simulink model "Digital Protection - Instantaneous Overcurrent Element SLG Simulink"  (R2024b)
settings: Solver=ode4  StartTime=0.0  StopTime=1  FixedStep=1e-5  RelTol=1e-4
undefined symbols (not defined in the file): D1, Delta, dspblkCoreblockFVToolHelper, gcbh, rvar
libraries: spsThreePhaseBreakerLib x6, dspfdesign x6, powerlib_extras x6, simulink_extras x6, spsLoadFlowBusLib x4, spsThreePhaseVIMeasurementLib x4, spsDistributedParametersLineLib x3, spsThreePhaseSeriesRLCLoadLib x3, spsGroundLib x3, spsThreePhaseSeriesRLCBranchLib x2, spsSeriesRLCBranchLib x2, spsThreePhaseTransformerTwoWindingsLib x1
(part 1 of 2)
settings Model: Creator=The MathWorks, Inc.  LastModifiedBy=ECDG
settings SolverCC: AlgebraicLoopSolver=TrustRegion  EnableFixedStepZeroCrossing=on
settings DataIOCC: SaveFormat=Array  ReturnWorkspaceOutputs=off  SignalLoggingName=sigsOut
settings OptimizationCC: BlockReduction=off  BooleanDataType=off  ReuseModelBlockBuffer=off  ExpressionDepthLimit=2147483647  InitFltsAndDblsToZero=on  LifeSpan=inf
settings DebuggingCC: UnderspecifiedInitializationDetection=Classic  MergeDetectMultiDrivingBlocksExec=none  CheckExecutionContextPreStartOutputMsg=on  SignalResolutionControl=TryResolveAllWithWarning  MultiTaskDSMMsg=warning  MultiTaskCondExecSysMsg=none  FcnCallInpInsideContextMsg=warning  UnconnectedInputMsg=warning  UnconnectedOutputMsg=warning  UnconnectedLineMsg=warning  StateNameClashWarn=warning  SFUnexpectedBacktrackingDiag=warning  SFNoUnconditionalDefaultTransitionDiag=warning  SFExecutionAtInitializationDiag=none  ArithmeticOperatorsInVariantConditions=warning
settings HardwareCC: ProdBitPerPointer=32  ProdBitPerSizeT=32  ProdBitPerPtrDiffT=32  ProdLargestAtomicFloat=None  ProdIntDivRoundTo=Undefined  ProdEndianess=Unspecified  ProdWordSize=32  ProdHWDeviceType=32-bit Generic  TargetUnknown=on
settings ModelReferenceCC: EnableRefExpFcnMdlSchedulingChecks=on  PropagateSignalLabelsOutOfModel=off
settings SFSimCC: SimUseLocalCustomCode=off  CustomCodeUndefinedFunction=UseInterfaceOnly
settings RTWCC: RTWUseLocalCustomCode=off  GPUComputeCapability=3.5  DLArmComputeVersion=19.05
settings CodeAppCC: StateflowObjectComments=on
settings GRTTargetCC: TargetLangStandard=C89/C90 (ANSI)  CombineOutputUpdateFcns=off  GRTInterface=on
settings ConfigComp: CovMetricSettings=dw  CovSaveCumulativeToWorkspaceVar=on  CovSaveSingleToWorkspaceVar=on  CovExternalEMLEnable=off  CovSFcnEnable=off
settings SimscapeCC: SimscapeNormalizeSystem=off

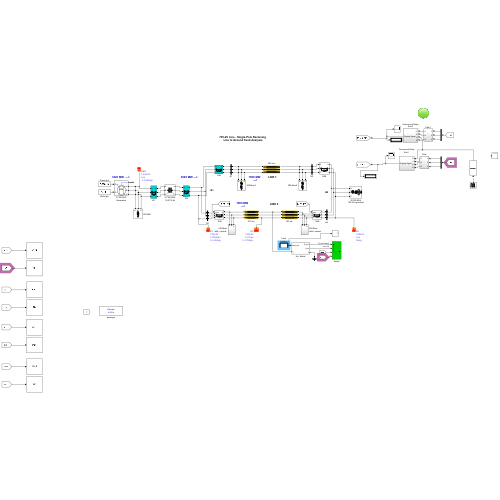
[thumbnail: Simulink's stored preview of the top-level diagram]
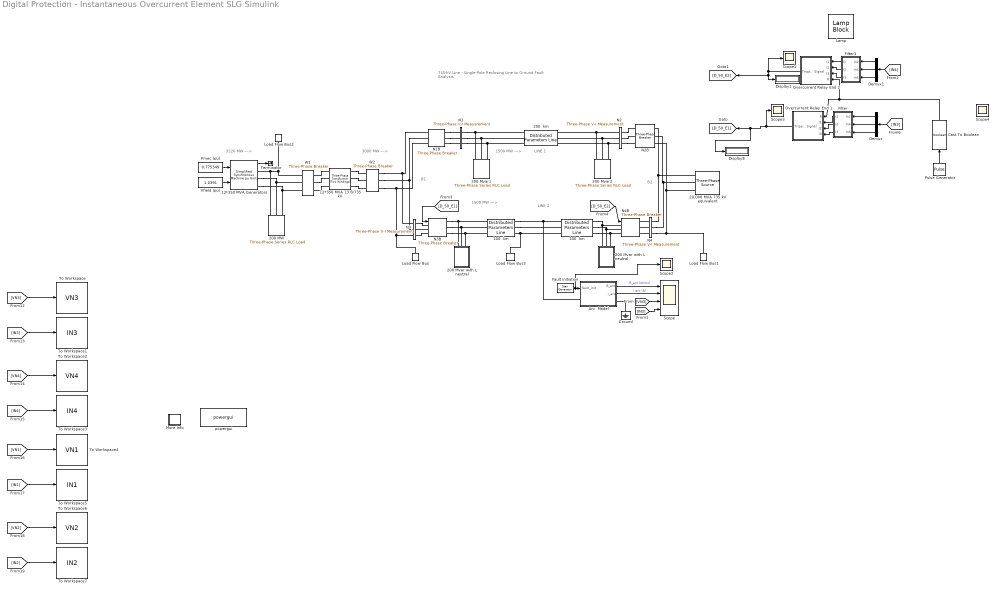
== system Digital Protection - Instantaneous Overcurrent Element SLG Simulink ==
  note: 735-kV Line - Single-Pole Reclosing
      | Line to Ground Fault Analysis
  note: LINE 1
  note: LINE 2
  note: B1
  note: B2
  note: 1500 MW
      |   --->
  note: 1500 MW
      |   --->
  note: 3220 MW --->
  note: 3000 MW --->
  "  N3B" : spsThreePhaseBreakerLib/Three-Phase Breaker  InitialState=closed  SwitchA=on  SwitchB=off  SwitchC=off  SwitchTimes=[0.4]  External=on  BreakerResistance=0.001  SnubberResistance=1e5  SnubberCapacitance=inf  Measurements=None
      settings: AttributesFormatString=\n
  "  N4B" : spsThreePhaseBreakerLib/Three-Phase Breaker  InitialState=closed  SwitchA=on  SwitchB=off  SwitchC=off  SwitchTimes=[0.2]  External=on  BreakerResistance=0.001  SnubberResistance=1e5  SnubberCapacitance=inf  Measurements=None
      settings: AttributesFormatString=\n
  " N1B" : spsThreePhaseBreakerLib/Three-Phase Breaker  InitialState=closed  SwitchA=off  SwitchB=off  SwitchC=off  SwitchTimes="[4/60  34/60]"  External=off  BreakerResistance=0.001  SnubberResistance=1e5  SnubberCapacitance=inf  Measurements=None
      settings: AttributesFormatString=\n
  " W2" : spsThreePhaseBreakerLib/Three-Phase Breaker  InitialState=closed  SwitchA=off  SwitchB=off  SwitchC=off  SwitchTimes="[4/60  34/60]"  External=off  BreakerResistance=0.001  SnubberResistance=1e5  SnubberCapacitance=inf  Measurements=Breaker voltages and currents
      settings: AttributesFormatString=\n
  "100  km " : spsDistributedParametersLineLib/Distributed Parameters Line  Phases=3  Length=100  Frequency=60  Resistance=[0.01165 0.2676]  Inductance="[0.8679e-3  3.008e-3]"  Capacitance="[13.41e-9  8.57e-9]"  x1=[-0.00051 -3.77922811047225e-08 0 0;-0.0005 -3.76584518295274e-08 0 0;-0.00049 -3.75240873443748e-08 0 0;-0.00048 -3.73891895588812e-08 0 0;-0.00047 -3.72537603902428e-08 0 0;-0.00046 -3.71178017632078e-08 0 0;-0.00045 -3.69813156100494e-08 0 0;-0.00044 -3.68443038705378e-08 0 0;-0.00043 -3.67067684919131e-08 0 0;-0.00042 -3.65687114288575e-08 0 0;-0.00041 -3.64301346434675e-08 0 0;-0.0004 -3.6291040105226e-08 0 0;-0.00039 -3.61514297909741e-08 0 0;-0.00038 -3.60113056848835e-08 0 0;-0.00037 -3.58706697784279e-08 0 0;-0.00036 -3.57295240703548e-08 0 0;-0.00035 -3.55878705666572e-08 395978.931287506 -613583.344384587;-0.00034 -3.54457112805449e-08 398289.270800667 -612086.189257274;-0.00033 -3.53030482324161e-08 400593.949741675 -610580.335030357;-0.00032 -3.51598834498283e-08 402892.93535594 -609065.803105355;-0.00031 -3.50162189674702e-08 405186.194969788 -607542.615007121;-0.0003 -3.4872056827132e-08 407473.695990923 -606010.792383529;-0.00029 -3.47273990776767e-08 409755.405908894 -604470.35700517;-0.00028 -3.45822477750113e-08 412031.292295551 -602921.330765038;-0.00027 -3.4436604982057e-08 414301.32280551 -601363.735678227;-0.00026 -3.42904727687203e-08 416565.465176615 -599797.593881611;-0.00025 -3.41438532118635e-08 418823.687230389 -598222.92763353;-0.00024 -3.39967483952749e-08 421075.9568725 -596639.759313478;-0.00023 -3.38491604096396e-08 423322.242093209 -595048.11142178;-0.00022 -3.37010913525096e-08 425562.510967832 -593448.006579278;-0.00021 -3.35525433282739e-08 427796.73165719 -591839.467527001;-0.0002 -3.34035184481288e-08 430024.87240806 -590222.517125851;-0.00019 -3.32540188300477e-08 432246.901553632 -588597.178356272;-0.00018 -3.3104046598751e-08 434462.787513951 -586963.474317926;-0.00017 -3.29536038856763e-08 436672.498796374 -585321.428229363;-0.00016 -3.28026928289473e-08 438876.003996012 -583671.063427693;-0.00015 -3.26513155733443e-08 441073.271796179 -582012.403368252;-0.00014 -3.24994742702731e-08 443264.270968836 -580345.471624272;-0.00013 -3.23471710777348e-08 445448.970375035 -578670.291886542;-0.00012 -3.21944081602949e-08 447627.338965361 -576986.887963075;-0.00011 -3.20411876890525e-08 449799.345780374 -575295.283778767;-0.0001 -3.18875118416097e-08 451964.959951051 -573595.503375057;-9e-05 -3.17333828020404e-08 454124.15069922 -571887.570909587;-8e-05 -3.15788027608595e-08 456276.887338002 -570171.510655858;-7e-05 -3.14237739149916e-08 458423.139272243 -568447.347002886;-6e-05 -3.12682984677396e-08 460562.875998953 -566715.104454851;-5e-05 -3.11123786287539e-08 462696.067107737 -564974.807630755;-4e-05 -3.09560166140004e-08 464822.682281227 -563226.481264068;-3e-05 -3.07992146457295e-08 466942.691295515 -561470.150202377;-2e-05 -3.06419749524443e-08 469056.064020578 -559705.839407035;-1e-05 -3.04842997688688e-08 471162.770420715 -557933.573952803]  x2=[-0.00051 -2.56040253138392e-08 0 0;-0.0005 -2.55064962507539e-08 0 0;-0.00049 -2.54086046838981e-08 0 0;-0.00048 -2.53103520045277e-08 0 0;-0.00047 -2.52117396090307e-08 0 0;-0.00046 -2.51127688989075e-08 0 0;-0.00045 -2.5013441280751e-08 0 0;-0.00044 -2.49137581662265e-08 0 0;-0.00043 -2.48137209720518e-08 0 0;-0.00042 -2.47133311199767e-08 0 0;-0.00041 -2.46125900367634e-08 0 0;-0.0004 -2.45114991541655e-08 0 0;-0.00039 -2.44100599089083e-08 0 0;-0.00038 -2.4308273742668e-08 0 0;-0.00037 -2.42061421020513e-08 0 0;-0.00036 -2.41036664385749e-08 0 0;-0.00035 -2.40008482086449e-08 340840.176223379 -651975.861370538;-0.00034 -2.38976888735358e-08 343295.642553621 -650686.299268294;-0.00033 -2.37941898993701e-08 345746.229892895 -649387.48947344;-0.00032 -2.36903527570974e-08 348191.903412932 -648079.450444938;-0.00031 -2.35861789224733e-08 350632.628355296 -646762.200772918;-0.0003 -2.34816698760386e-08 353068.370031884 -645435.759178413;-0.00029 -2.33768271030981e-08 355499.093825416 -644100.144513095;-0.00028 -2.32716520936998e-08 357924.765189925 -642755.375759005;-0.00027 -2.31661463426133e-08 360345.349651252 -641401.472028282;-0.00026 -2.30603113493089e-08 362760.812807534 -640038.452562896;-0.00025 -2.29541486179361e-08 365171.120329694 -638666.336734371;-0.00024 -2.28476596573023e-08 367576.237961925 -637285.14404351;-0.00023 -2.27408459808514e-08 369976.131522183 -635894.894120118;-0.00022 -2.26337091066421e-08 372370.766902668 -634495.606722723;-0.00021 -2.25262505573265e-08 374760.110070311 -633087.301738298;-0.0002 -2.24184718601286e-08 377144.127067255 -631669.999181973;-0.00019 -2.23103745468221e-08 379522.784011344 -630243.719196755;-0.00018 -2.22019601537092e-08 381896.047096597 -628808.482053238;-0.00017 -2.20932302215983e-08 384263.882593691 -627364.308149322;-0.00016 -2.19841862957825e-08 386626.256850443 -625911.218009912;-0.00015 -2.18748299260173e-08 388983.136292286 -624449.232286636;-0.00014 -2.17651626664989e-08 391334.487422747 -622978.371757548;-0.00013 -2.16551860758416e-08 393680.27682392 -621498.657326831;-0.00012 -2.15449017170563e-08 396020.471156946 -620010.110024504;-0.00011 -2.14343111575279e-08 398355.037162483 -618512.751006117;-0.0001 -2.13234159689929e-08 400683.941661182 -617006.601552457;-9e-05 -2.12122177275176e-08 403007.151554153 -615491.683069241;-8e-05 -2.1100718013475e-08 405324.633823443 -613968.017086816;-7e-05 -2.09889184115228e-08 407636.355532497 -612435.625259845;-6e-05 -2.0876820510581e-08 409942.283826634 -610894.529367011;-5e-05 -2.07644259038087e-08 412242.385933509 -609344.751310696;-4e-05 -2.06517361885822e-08 414536.629163579 -607786.313116677;-3e-05 -2.05387529664718e-08 416824.980910569 -606219.23693381;-2e-05 -2.0425477843219e-08 419107.408651936 -604643.545033717;-1e-05 -2.03119124287142e-08 421383.87994933 -603059.259810467]  x3=[-0.00051 3.42496863435419e-11 0 0;-0.0005 3.47494854439e-11 0 0;-0.00049 3.52487906771517e-11 0 0;-0.00048 3.57475949470645e-11 0 0;-0.00047 3.62458911645256e-11 0 0;-0.00046 3.67436722476428e-11 0 0;-0.00045 3.72409311218451e-11 0 0;-0.00044 3.77376607199831e-11 0 0;-0.00043 3.82338539824298e-11 0 0;-0.00042 3.87295038571805e-11 0 0;-0.00041 3.92246032999535e-11 0 0;-0.0004 3.97191452742897e-11 0 0;-0.00039 4.0213122751653e-11 0 0;-0.00038 4.07065287115301e-11 0 0;-0.00037 4.119935614153e-11 0 0;-0.00036 4.16915980374842e-11 0 0;-0.00035 4.21832474035457e-11 164.000176487801 -861.324068209358;-0.00034 4.26742972522888e-11 167.246078376088 -860.699738770174;-0.00033 4.31647406048081e-11 170.4896033274 -860.063176882539;-0.00032 4.36545704908181e-11 173.73070524407 -859.414391593406;-0.00031 4.41437799487517e-11 176.969338062865 -858.75339212345;-0.0003 4.46323620258598e-11 180.205455755643 -858.080187866937;-0.00029 4.51203097783096e-11 183.439012330009 -857.39478839159;-0.00028 4.56076162712833e-11 186.669961829966 -856.697203438451;-0.00027 4.60942745790771e-11 189.898258336571 -855.987442921748;-0.00026 4.65802777851993e-11 193.123855968584 -855.265516928748;-0.00025 4.70656189824684e-11 196.346708883124 -854.531435719618;-0.00024 4.75502912731118e-11 199.566771276315 -853.785209727276;-0.00023 4.80342877688633e-11 202.783997383945 -853.026849557246;-0.00022 4.85176015910616e-11 205.998341482108 -852.256365987505;-0.00021 4.90002258707472e-11 209.209757887861 -851.473769968328;-0.0002 4.9482153748761e-11 212.418200959867 -850.679072622139;-0.00019 4.9963378375841e-11 215.623625099048 -849.872285243346;-0.00018 5.044389291272e-11 218.825984749233 -849.053419298182;-0.00017 5.0923690530223e-11 222.025234397802 -848.222486424545;-0.00016 5.14027644093637e-11 225.221328576336 -847.379498431832;-0.00015 5.18811077414418e-11 228.414221861263 -846.524467300767;-0.00014 5.23587137281398e-11 231.603868874501 -845.657405183235;-0.00013 5.28355755816194e-11 234.790224284105 -844.778324402109;-0.00012 5.33116865246182e-11 237.973242804914 -843.887237451071;-0.00011 5.37870397905458e-11 241.152879199187 -842.98415699444;-0.0001 5.426162862358e-11 244.329088277253 -842.069095866989;-9e-05 5.47354462787631e-11 247.501824898151 -841.142067073761;-8e-05 5.52084860220974e-11 250.671043970271 -840.203083789887;-7e-05 5.56807411306411e-11 253.836700451994 -839.252159360399;-6e-05 5.61522048926036e-11 256.998749352335 -838.289307300037;-5e-05 5.66228706074415e-11 260.15714573158 -837.314541293061;-4e-05 5.70927315859529e-11 263.311844701925 -836.327875193052;-3e-05 5.75617811503735e-11 266.462801428114 -835.329323022721;-2e-05 5.80300126344706e-11 269.609971128078 -834.318898973704;-1e-05 5.84974193836385e-11 272.753309073569 -833.296617406363]  x4=[-0.00051 -1.51149043943084e-10 0 0;-0.0005 -1.51308414634417e-10 0 0;-0.00049 -1.51465634898256e-10 0 0;-0.00048 -1.51620702500153e-10 0 0;-0.00047 -1.51773615236255e-10 0 0;-0.00046 -1.51924370933332e-10 0 0;-0.00045 -1.52072967448813e-10 0 0;-0.00044 -1.52219402670812e-10 0 0;-0.00043 -1.52363674518161e-10 0 0;-0.00042 -1.52505780940437e-10 0 0;-0.00041 -1.52645719917994e-10 0 0;-0.0004 -1.52783489461988e-10 0 0;-0.00039 -1.52919087614411e-10 0 0;-0.00038 -1.5305251244811e-10 0 0;-0.00037 -1.53183762066826e-10 0 0;-0.00036 -1.53312834605209e-10 0 0;-0.00035 -1.53439728228854e-10 2402.72875516981 -4282.32087607898;-0.00034 -1.53564441134322e-10 2418.85568395253 -4273.23238215375;-0.00033 -1.53686971549165e-10 2434.94823544183 -4264.08315613756;-0.00032 -1.53807317731955e-10 2451.00618092693 -4254.87332806114;-0.00031 -1.53925477972307e-10 2467.02929218889 -4245.60302881654;-0.0003 -1.54041450590902e-10 2483.01734150382 -4236.27239015525;-0.00029 -1.54155233939513e-10 2498.97010164616 -4226.88154468627;-0.00028 -1.54266826401026e-10 2514.88734589186 -4217.43062587432;-0.00027 -1.54376226389465e-10 2530.76884802167 -4207.91976803788;-0.00026 -1.54483432350015e-10 2546.61438232428 -4198.34910634727;-0.00025 -1.54588442759041e-10 2562.42372359957 -4188.7187768228;-0.00024 -1.54691256124114e-10 2578.19664716181 -4179.02891633276;-0.00023 -1.54791870984027e-10 2593.93292884284 -4169.27966259151;-0.00022 -1.5489028590882e-10 2609.63234499527 -4159.47115415754;-0.00021 -1.54986499499801e-10 2625.29467249564 -4149.60353043146;-0.0002 -1.5508051038956e-10 2640.91968874761 -4139.67693165403;-0.00019 -1.55172317241994e-10 2656.50717168512 -4129.69149890421;-0.00018 -1.55261918752327e-10 2672.05689977552 -4119.6473740971;-0.00017 -1.5534931364712e-10 2687.56865202276 -4109.54469998194;-0.00016 -1.554345006843e-10 2703.04220797051 -4099.3836201401;-0.00015 -1.55517478653171e-10 2718.47734770529 -4089.16427898301;-0.00014 -1.5559824637443e-10 2733.87385185959 -4078.88682175012;-0.00013 -1.55676802700192e-10 2749.23150161502 -4068.55139450686;-0.00012 -1.55753146513995e-10 2764.55007870536 -4058.15814414253;-0.00011 -1.55827276730826e-10 2779.82936541975 -4047.70721836821;-0.0001 -1.55899192297131e-10 2795.06914460568 -4037.1987657147;-9e-05 -1.55968892190829e-10 2810.26919967217 -4026.63293553036;-8e-05 -1.56036375421331e-10 2825.42931459278 -4016.00987797904;-7e-05 -1.56101641029551e-10 2840.54927390874 -4005.32974403789;-6e-05 -1.5616468808792e-10 2855.62886273193 -3994.59268549527;-5e-05 -1.562255157004e-10 2870.66786674804 -3983.79885494852;-4e-05 -1.56284123002496e-10 2885.66607221953 -3972.9484058019;-3e-05 -1.56340509161269e-10 2900.62326598869 -3962.04149226428;-2e-05 -1.56394673375345e-10 2915.5392354807 -3951.07826934705;-1e-05 -1.56446614874933e-10 2930.41376870661 -3940.05889286189]  x5=0.000507725910309884  V1=ones(3,3)  V2=ones(3,3)  I1=ones(3,3)  I2=ones(3,3)  nHarmo=1  Measurements=None  Decoupling=off  VsMag0=0  VrMag0=0  VsAngle0=0  VrAngle0=0  IsMag0=0  IrMag0=0  IsAngle0=0  IrAngle0=0
      settings: AttributesFormatString=\n
  "100  km  " : spsDistributedParametersLineLib/Distributed Parameters Line  Phases=3  Length=100  Frequency=60  Resistance=[0.01165 0.2676]  Inductance="[0.8679e-3  3.008e-3]"  Capacitance="[13.41e-9  8.57e-9]"  x1=[-0.00051 -2.56040253138392e-08 0 0;-0.0005 -2.55064962507539e-08 0 0;-0.00049 -2.54086046838981e-08 0 0;-0.00048 -2.53103520045277e-08 0 0;-0.00047 -2.52117396090307e-08 0 0;-0.00046 -2.51127688989075e-08 0 0;-0.00045 -2.5013441280751e-08 0 0;-0.00044 -2.49137581662265e-08 0 0;-0.00043 -2.48137209720518e-08 0 0;-0.00042 -2.47133311199767e-08 0 0;-0.00041 -2.46125900367634e-08 0 0;-0.0004 -2.45114991541655e-08 0 0;-0.00039 -2.44100599089083e-08 0 0;-0.00038 -2.4308273742668e-08 0 0;-0.00037 -2.42061421020513e-08 0 0;-0.00036 -2.41036664385749e-08 0 0;-0.00035 -2.40008482086449e-08 340840.176223379 -651975.861370538;-0.00034 -2.38976888735358e-08 343295.642553621 -650686.299268294;-0.00033 -2.37941898993701e-08 345746.229892895 -649387.48947344;-0.00032 -2.36903527570974e-08 348191.903412932 -648079.450444938;-0.00031 -2.35861789224733e-08 350632.628355296 -646762.200772918;-0.0003 -2.34816698760386e-08 353068.370031884 -645435.759178413;-0.00029 -2.33768271030981e-08 355499.093825416 -644100.144513095;-0.00028 -2.32716520936998e-08 357924.765189925 -642755.375759005;-0.00027 -2.31661463426133e-08 360345.349651252 -641401.472028282;-0.00026 -2.30603113493089e-08 362760.812807534 -640038.452562896;-0.00025 -2.29541486179361e-08 365171.120329694 -638666.336734371;-0.00024 -2.28476596573023e-08 367576.237961925 -637285.14404351;-0.00023 -2.27408459808514e-08 369976.131522183 -635894.894120118;-0.00022 -2.26337091066421e-08 372370.766902668 -634495.606722723;-0.00021 -2.25262505573265e-08 374760.110070311 -633087.301738298;-0.0002 -2.24184718601286e-08 377144.127067255 -631669.999181973;-0.00019 -2.23103745468221e-08 379522.784011344 -630243.719196755;-0.00018 -2.22019601537092e-08 381896.047096597 -628808.482053238;-0.00017 -2.20932302215983e-08 384263.882593691 -627364.308149322;-0.00016 -2.19841862957825e-08 386626.256850443 -625911.218009912;-0.00015 -2.18748299260173e-08 388983.136292286 -624449.232286636;-0.00014 -2.17651626664989e-08 391334.487422747 -622978.371757548;-0.00013 -2.16551860758416e-08 393680.27682392 -621498.657326831;-0.00012 -2.15449017170563e-08 396020.471156946 -620010.110024504;-0.00011 -2.14343111575279e-08 398355.037162483 -618512.751006117;-0.0001 -2.13234159689929e-08 400683.941661182 -617006.601552457;-9e-05 -2.12122177275176e-08 403007.151554153 -615491.683069241;-8e-05 -2.1100718013475e-08 405324.633823443 -613968.017086816;-7e-05 -2.09889184115228e-08 407636.355532497 -612435.625259845;-6e-05 -2.0876820510581e-08 409942.283826634 -610894.529367011;-5e-05 -2.07644259038087e-08 412242.385933509 -609344.751310696;-4e-05 -2.06517361885822e-08 414536.629163579 -607786.313116677;-3e-05 -2.05387529664718e-08 416824.980910569 -606219.23693381;-2e-05 -2.0425477843219e-08 419107.408651936 -604643.545033717;-1e-05 -2.03119124287142e-08 421383.87994933 -603059.259810467]  x2=[-0.00051 -1.18539215505797e-08 0 0;-0.0005 -1.17942402554783e-08 0 0;-0.00049 -1.17343913381163e-08 0 0;-0.00048 -1.16743756490792e-08 0 0;-0.00047 -1.16141940413229e-08 0 0;-0.00046 -1.15538473701611e-08 0 0;-0.00045 -1.14933364932537e-08 0 0;-0.00044 -1.14326622705942e-08 0 0;-0.00043 -1.13718255644975e-08 0 0;-0.00042 -1.1310827239588e-08 0 0;-0.00041 -1.12496681627868e-08 0 0;-0.0004 -1.11883492032999e-08 0 0;-0.00039 -1.11268712326053e-08 0 0;-0.00038 -1.10652351244411e-08 0 0;-0.00037 -1.10034417547928e-08 0 0;-0.00036 -1.0941492001881e-08 0 0;-0.00035 -1.08793867461488e-08 280454.28762092 -679398.727325685;-0.00034 -1.08171268702493e-08 283013.563488485 -678336.617298876;-0.00033 -1.07547132590333e-08 285568.817106861 -677264.866607234;-0.00032 -1.06921467995362e-08 288120.012160238 -676183.490482708;-0.00031 -1.0629428380966e-08 290667.112390487 -675092.504294046;-0.0003 -1.05665588946902e-08 293210.081597675 -673991.923546578;-0.00029 -1.05035392342234e-08 295748.883640582 -672881.763881991;-0.00028 -1.04403702952144e-08 298283.482437211 -671762.041078112;-0.00027 -1.03770529754337e-08 300813.841965302 -670632.77104868;-0.00026 -1.03135881747606e-08 303339.926262846 -669493.969843123;-0.00025 -1.02499767951703e-08 305861.699428593 -668345.653646326;-0.00024 -1.01862197407214e-08 308379.125622564 -667187.838778404;-0.00023 -1.01223179175427e-08 310892.169066562 -666020.541694469;-0.00022 -1.00582722338206e-08 313400.794044676 -664843.778984397;-0.00021 -9.99408359978607e-09 315904.964903792 -663657.56737259;-0.0002 -9.92975292770159e-09 318404.6460541 -662461.923717741;-0.00019 -9.86528113184844e-09 320899.801969597 -661256.865012593;-0.00018 -9.80066912851356e-09 323390.397188594 -660042.408383698;-0.00017 -9.73591783597653e-09 325876.396314221 -658818.571091172;-0.00016 -9.67102817449654e-09 328357.764014927 -657585.370528453;-0.00015 -9.60600106629932e-09 330834.465024985 -656342.824222049;-0.00014 -9.54083743556401e-09 333306.464144991 -655090.949831296;-0.00013 -9.47553820841005e-09 335773.726242367 -653829.765148098;-0.00012 -9.410104312884e-09 338236.216251855 -652559.288096681;-0.00011 -9.34453667894634e-09 340693.899176022 -651279.536733337;-0.0001 -9.2788362384583e-09 343146.740085755 -649990.529246166;-9e-05 -9.21300392516855e-09 345594.704120754 -648692.283954816;-8e-05 -9.1470406747e-09 348037.756490031 -647384.819310228;-7e-05 -9.08094742453643e-09 350475.862472406 -646068.153894367;-6e-05 -9.01472511400924e-09 352908.987416994 -644742.306419965;-5e-05 -8.94837468428403e-09 355337.096743706 -643407.295730247;-4e-05 -8.88189707834729e-09 357760.155943732 -642063.140798672;-3e-05 -8.81529324099293e-09 360178.130580038 -640709.860728656;-2e-05 -8.74856411880893e-09 362590.986287852 -639347.474753305;-1e-05 -8.6817106601638e-09 364998.688775155 -637976.002235138]  x3=[-0.00051 6.32300703573828e-11 0 0;-0.0005 6.37254256125662e-11 0 0;-0.00049 6.42198751883951e-11 0 0;-0.00048 6.47134120576465e-11 0 0;-0.00047 6.52060292060691e-11 0 0;-0.00046 6.56977196324828e-11 0 0;-0.00045 6.61884763488782e-11 0 0;-0.00044 6.66782923805162e-11 0 0;-0.00043 6.71671607660268e-11 0 0;-0.00042 6.76550745575079e-11 0 0;-0.00041 6.81420268206248e-11 0 0;-0.0004 6.86280106347078e-11 0 0;-0.00039 6.91130190928512e-11 0 0;-0.00038 6.95970453020112e-11 0 0;-0.00037 7.00800823831041e-11 0 0;-0.00036 7.05621234711037e-11 0 0;-0.00035 7.10431617151392e-11 267.626302043254 -825.665681968738;-0.00034 7.15231902785922e-11 270.737031817784 -824.650940062222;-0.00033 7.20022023391944e-11 273.843913819813 -823.624478040479;-0.00032 7.24801910891242e-11 276.946903893672 -822.586310491806;-0.00031 7.29571497351032e-11 280.045957939003 -821.536452170861;-0.0003 7.34330714984936e-11 283.141031911389 -820.474917998456;-0.00029 7.39079496153934e-11 286.232081822977 -819.401723061341;-0.00028 7.43817773367335e-11 289.319063743106 -818.316882611991;-0.00027 7.48545479283732e-11 292.40193379893 -817.22041206839;-0.00026 7.5326254671196e-11 295.480648176041 -816.112327013812;-0.00025 7.57968908612048e-11 298.555163119094 -814.992643196598;-0.00024 7.62664498096176e-11 301.625434932426 -813.861376529934;-0.00023 7.67349248429625e-11 304.691419980678 -812.718543091623;-0.00022 7.72023093031721e-11 307.753074689415 -811.564159123858;-0.00021 7.76685965476789e-11 310.810355545749 -810.39824103299;-0.0002 7.81337799495088e-11 313.863219098949 -809.220805389296;-0.00019 7.85978528973762e-11 316.911621961069 -808.031868926743;-0.00018 7.90608087957771e-11 319.955520807555 -806.83144854275;-0.00017 7.95226410650835e-11 322.994872377866 -805.619561297947;-0.00016 7.99833431416366e-11 326.029633476091 -804.396224415936;-0.00015 8.04429084778401e-11 329.059760971555 -803.16145528304;-0.00014 8.09013305422533e-11 332.085211799441 -801.915271448062;-0.00013 8.1358602819684e-11 335.105942961394 -800.657690622033;-0.00012 8.18147188112809e-11 338.12191152614 -799.388730677961;-0.00011 8.22696720346262e-11 341.133074630088 -798.108409650574;-0.0001 8.27234560238275e-11 344.139389477945 -796.816745736069;-9e-05 8.317606432961e-11 347.140813343324 -795.513757291849;-8e-05 8.36274905194076e-11 350.137303569347 -794.199462836264;-7e-05 8.40777281774551e-11 353.128817569255 -792.873881048347;-6e-05 8.45267709048787e-11 356.115312827014 -791.537030767551;-5e-05 8.49746123197872e-11 359.096746897913 -790.188930993475;-4e-05 8.5421246057363e-11 362.073077409177 -788.829600885603;-3e-05 8.58666657699519e-11 365.044262060561 -787.459059763024;-2e-05 8.63108651271539e-11 368.010258624953 -786.077327104161;-1e-05 8.67538378159128e-11 370.971024948977 -784.684422546493]  x4=[-0.00051 -1.32243517909503e-10 0 0;-0.0005 -1.3251038312282e-10 0 0;-0.00049 -1.32775365070281e-10 0 0;-0.00048 -1.33038459985904e-10 0 0;-0.00047 -1.3329966413053e-10 0 0;-0.00046 -1.3355897379187e-10 0 0;-0.00045 -1.33816385284558e-10 0 0;-0.00044 -1.34071894950208e-10 0 0;-0.00043 -1.34325499157462e-10 0 0;-0.00042 -1.34577194302042e-10 0 0;-0.00041 -1.34826976806805e-10 0 0;-0.0004 -1.35074843121786e-10 0 0;-0.00039 -1.35320789724258e-10 0 0;-0.00038 -1.35564813118775e-10 0 0;-0.00037 -1.35806909837224e-10 0 0;-0.00036 -1.36047076438875e-10 0 0;-0.00035 -1.36285309510428e-10 1829.93758676739 -4546.62282566466;-0.00034 -1.36521605666066e-10 1847.06497615061 -4539.69181135784;-0.00033 -1.36755961547495e-10 1864.16611465204 -4532.69627798175;-0.00032 -1.36988373824001e-10 1881.24075922663 -4525.63632495841;-0.00031 -1.3721883919249e-10 1898.2886672059 -4518.51205262537;-0.0003 -1.3744735437754e-10 1915.30959630133 -4511.32356223431;-0.00029 -1.37673916131444e-10 1932.30330460786 -4504.0709559496;-0.00028 -1.37898521234257e-10 1949.26955060726 -4496.75433684681;-0.00027 -1.38121166493845e-10 1966.20809317163 -4489.37380891131;-0.00026 -1.38341848745924e-10 1983.11869156678 -4481.92947703673;-0.00025 -1.38560564854113e-10 2000.00110545568 -4474.42144702351;-0.00024 -1.38777311709971e-10 2016.85509490187 -4466.84982557737;-0.00023 -1.38992086233045e-10 2033.68042037283 -4459.21472030781;-0.00022 -1.39204885370913e-10 2050.47684274345 -4451.51623972658;-0.00021 -1.3941570609923e-10 2067.2441232994 -4443.75449324613;-0.0002 -1.39624545421766e-10 2083.98202374051 -4435.92959117806;-0.00019 -1.39831400370452e-10 2100.69030618415 -4428.04164473154;-0.00018 -1.40036268005421e-10 2117.36873316865 -4420.09076601176;-0.00017 -1.4023914541505e-10 2134.01706765664 -4412.0770680183;-0.00016 -1.40440029716003e-10 2150.63507303845 -4404.00066464355;-0.00015 -1.40638918053269e-10 2167.22251313542 -4395.86167067107;-0.00014 -1.40835807600205e-10 2183.77915220333 -4387.66020177399;-0.00013 -1.41030695558574e-10 2200.30475493567 -4379.39637451333;-0.00012 -1.41223579158586e-10 2216.79908646706 -4371.07030633638;-0.00011 -1.4141445565894e-10 2233.26191237654 -4362.68211557498;-0.0001 -1.41603322346857e-10 2249.6929986909 -4354.2319214439;-9e-05 -1.41790176538124e-10 2266.09211188805 -4345.71984403911;-8e-05 -1.41975015577129e-10 2282.45901890028 -4337.14600433605;-7e-05 -1.421578368369e-10 2298.79348711761 -4328.51052418798;-6e-05 -1.42338637719143e-10 2315.0952843911 -4319.81352632418;-5e-05 -1.42517415654276e-10 2331.36417903613 -4311.05513434824;-4e-05 -1.4269416810147e-10 2347.59993983568 -4302.23547273629;-3e-05 -1.42868892548681e-10 2363.80233604367 -4293.35466683526;-2e-05 -1.43041586512687e-10 2379.97113738817 -4284.41284286105;-1e-05 -1.43212247539126e-10 2396.10611407473 -4275.41012789677]  x5=0.000507725910309884  V1=ones(3,3)  V2=ones(3,3)  I1=ones(3,3)  I2=ones(3,3)  nHarmo=1  Measurements=None  Decoupling=off  VsMag0=0  VrMag0=0  VsAngle0=0  VrAngle0=0  IsMag0=0  IrMag0=0  IsAngle0=0  IrAngle0=0
      settings: AttributesFormatString=\n
  12*350 MVA 13.8/735 kV : spsThreePhaseTransformerTwoWindingsLib/Three-Phase Transformer (Two Windings)  Winding1Connection=Delta (D1)  Winding2Connection=Yg  CoreType=Three single-phase transformers  SetSaturation=off  Hysteresis=off  DataFile='hysteresis'  SetInitialFlux=off  Measurements=None  UNITS=pu  NominalPower=[ 12*350e6 , 60 ]  Winding1=[ 13.8e3 , 0.002 , 0.08 ]  Winding2=[ 735e3 , 0.002 , 0.08 ]  Rm=500  Lm=500  L0=0.5  Saturation=[ 0,0 ; 0.0024,1.2 ; 1.0,1.52 ]  InitialFluxes=[ 0.8 , -0.8 , 0.7 ]  BreakLoop=off  DiscreteSolver=Trapezoidal iterative  DataType=off  TransfoNumber=0
  12*350 MVA Generators : spsSimplifiedSynchronousMachinepuUnitsLib/Simplified Synchronous Machine pu Units  ConnectionType=3-wire Y  MechanicalLoad=Mechanical power Pm  MeasurementBus=off  NominalParameters=[ 12*350e6,13.8e3,60 ]  Mechanical=[ inf,0,2 ]  InternalRL=[ 0.22/15, 0.22 ]  InitialConditions=[0 -3.66888 0.76939 0.76939 0.76939 -17.7796 -137.78 102.22 ]  IterativeDiscreteModel=Trapezoidal non iterative  TsBlock=-1  TsPowergui=0  LoadFlowParameters=[1 3000000000 0 0 0]  Units=0  BusType=PV  Pref=3220e+006  Qref=0  Qmin=-Inf  Qmax=Inf  PLF=0  QLF=0
      settings: AttributesFormatString=\n
  20,000 MVA 735 kV equivalent : spsThreePhaseSourceLib/Three-Phase Source  InternalConnection=Yg  VoltagePhases=off  Voltage=(735000)*1.01317  PhaseAngle=-8.5536  Voltage_phases=[25e3 25e3 25e3]/sqrt(3)  PhaseAngles_phases=[0 -120 +120]  Frequency=60  NonIdealSource=on  SpecifyImpedance=on  Resistance=735^2/20000/10  Inductance=735^2/20000/377  ShortCircuitLevel=20000e6  BaseVoltage=735e3  XRratio=10  BusType=swing  Pref=0  Qref=0  Prefabc=[10e3, 10e3, 10e3]  Qrefabc=[0, 0, 0]  Qmin=-Inf  Qmax=Inf
  200  km : spsDistributedParametersLineLib/Distributed Parameters Line  Phases=3  Length=200  Frequency=60  Resistance=[0.01165 0.2676]  Inductance="[0.8679e-3  3.008e-3]"  Capacitance="[13.41e-9  8.57e-9]"  x1=[-0.00102 -3.37976126828733e-08 0 0;-0.00101 -3.37486811324577e-08 0 0;-0.001 -3.36992699385804e-08 0 0;-0.00099 -3.36493798034838e-08 0 0;-0.00098 -3.3599011436217e-08 0 0;-0.00097 -3.35481655526262e-08 0 0;-0.00096 -3.34968428753438e-08 0 0;-0.00095 -3.34450441337788e-08 0 0;-0.00094 -3.33927700641058e-08 0 0;-0.00093 -3.33400214092551e-08 0 0;-0.00092 -3.32867989189019e-08 0 0;-0.00091 -3.32331033494555e-08 0 0;-0.0009 -3.31789354640489e-08 0 0;-0.00089 -3.31242960325276e-08 0 0;-0.00088 -3.30691858314389e-08 0 0;-0.00087 -3.30136056440206e-08 0 0;-0.00086 -3.29575562601904e-08 0 0;-0.00085 -3.2901038476534e-08 0 0;-0.00084 -3.28440530962943e-08 0 0;-0.00083 -3.27866009293595e-08 0 0;-0.00082 -3.27286827922523e-08 0 0;-0.00081 -3.26702995081174e-08 0 0;-0.0008 -3.26114519067107e-08 0 0;-0.00079 -3.25521408243867e-08 0 0;-0.00078 -3.24923671040873e-08 0 0;-0.00077 -3.24321315953293e-08 0 0;-0.00076 -3.23714351541927e-08 0 0;-0.00075 -3.23102786433081e-08 0 0;-0.00074 -3.22486629318451e-08 0 0;-0.00073 -3.21865888954992e-08 0 0;-0.00072 -3.212405741648e-08 0 0;-0.00071 -3.2061069383498e-08 0 0;-0.0007 -3.19976256917528e-08 0 0;-0.00069 -3.19337272429196e-08 314298.322581324 -659166.140545734;-0.00068 -3.18693749451368e-08 316781.086063076 -657976.588826017;-0.00067 -3.1804569712993e-08 319259.347384399 -656777.685802537;-0.00066 -3.1739312467514e-08 321733.071323713 -655569.448514361;-0.00065 -3.16736041361497e-08 324202.222723926 -654351.894133215;-0.00064 -3.16074456527609e-08 326666.76649293 -653125.039963243;-0.00063 -3.15408379576062e-08 329126.667604104 -651888.903440757;-0.00062 -3.14737819973283e-08 331581.891096808 -650643.502133993;-0.00061 -3.14062787249408e-08 334032.402076881 -649388.853742861;-0.0006 -3.13383290998146e-08 336478.165717138 -648124.976098692;-0.00059 -3.12699340876644e-08 338919.147257865 -646851.887163985;-0.00058 -3.12010946605346e-08 341355.312007309 -645569.60503215;-0.00057 -3.1131811796786e-08 343786.625342177 -644278.147927257;-0.00056 -3.10620864810812e-08 346213.052708127 -642977.534203768;-0.00055 -3.09919197043715e-08 348634.559620252 -641667.782346285;-0.00054 -3.0921312463882e-08 351051.111663581 -640348.910969279;-0.00053 -3.08502657630979e-08 353462.67449356 -639020.938816832;-0.00052 -3.07787806117501e-08 355869.213836543 -637683.884762369;-0.00051 -3.07068580258008e-08 358270.695490279 -636337.767808386;-0.0005 -3.06344990274291e-08 360667.085324398 -634982.607086186;-0.00049 -3.05617046450167e-08 363058.349280895 -633618.421855602;-0.00048 -3.04884759131327e-08 365444.453374618 -632245.231504726;-0.00047 -3.04148138725196e-08 367825.363693746 -630863.055549632;-0.00046 -3.03407195700781e-08 370201.046400272 -629471.913634099;-0.00045 -3.02661940588521e-08 372571.467730486 -628071.825529335;-0.00044 -3.01912383980141e-08 374936.593995455 -626662.811133689;-0.00043 -3.01158536528501e-08 377296.3915815 -625244.890472376;-0.00042 -3.0040040894744e-08 379650.826950672 -623818.083697186;-0.00041 -2.99638012011631e-08 381999.866641234 -622382.411086203;-0.0004 -2.9887135655642e-08 384343.477268133 -620937.893043511;-0.00039 -2.98100453477679e-08 386681.625523473 -619484.55009891;-0.00038 -2.97325313731648e-08 389014.278176993 -618022.402907619;-0.00037 -2.96545948334777e-08 391341.402076535 -616551.472249987;-0.00036 -2.95762368363574e-08 393662.964148517 -615071.779031195;-0.00035 -2.94974584954446e-08 395978.931398403 -613583.344280958;-0.00034 -2.94182609303537e-08 398289.270911173 -612086.189153228;-0.00033 -2.93386452666575e-08 400593.949851788 -610580.334925895;-0.00032 -2.92586126358709e-08 402892.935465658 -609065.80300048;-0.00031 -2.91781641754346e-08 405186.19507911 -607542.614901834;-0.0003 -2.90973010286993e-08 407473.696099848 -606010.792277831;-0.00029 -2.90160243449094e-08 409755.406017419 -604470.356899062;-0.00028 -2.89343352791865e-08 412031.292403675 -602921.330658523;-0.00027 -2.88522349925129e-08 414301.322913233 -601363.735571306;-0.00026 -2.87697246517155e-08 ...(+1661 chars)]  x2=[-0.00102 -7.63671288317374e-09 0 0;-0.00101 -7.64156246557535e-09 0 0;-0.001 -7.64630344445969e-09 0 0;-0.00099 -7.65093575244694e-09 0 0;-0.00098 -7.65545932370177e-09 0 0;-0.00097 -7.65987409393421e-09 0 0;-0.00096 -7.66418000040061e-09 0 0;-0.00095 -7.66837698190449e-09 0 0;-0.00094 -7.67246497879747e-09 0 0;-0.00093 -7.67644393298006e-09 0 0;-0.00092 -7.68031378790251e-09 0 0;-0.00091 -7.68407448856562e-09 0 0;-0.0009 -7.68772598152151e-09 0 0;-0.00089 -7.69126821487438e-09 0 0;-0.00088 -7.69470113828125e-09 0 0;-0.00087 -7.69802470295268e-09 0 0;-0.00086 -7.70123886165347e-09 0 0;-0.00085 -7.7043435687033e-09 0 0;-0.00084 -7.70733877997742e-09 0 0;-0.00083 -7.71022445290724e-09 0 0;-0.00082 -7.71300054648095e-09 0 0;-0.00081 -7.71566702124414e-09 0 0;-0.0008 -7.71822383930028e-09 0 0;-0.00079 -7.72067096431134e-09 0 0;-0.00078 -7.72300836149825e-09 0 0;-0.00077 -7.72523599764142e-09 0 0;-0.00076 -7.72735384108121e-09 0 0;-0.00075 -7.72936186171839e-09 0 0;-0.00074 -7.73126003101453e-09 0 0;-0.00073 -7.73304832199244e-09 0 0;-0.00072 -7.73472670923655e-09 0 0;-0.00071 -7.73629516889326e-09 0 0;-0.0007 -7.7377536786713e-09 0 0;-0.00069 -7.739102217842e-09 191308.512931951 -709674.654697389;-0.00068 -7.74034076723964e-09 193982.559946066 -708948.400100959;-0.00067 -7.7414693092617e-09 196653.850038623 -708212.069778503;-0.00066 -7.74248782786909e-09 199322.345244676 -707465.674194903;-0.00065 -7.7433963085864e-09 201988.007639002 -706709.223958095;-0.00064 -7.74419473850212e-09 204650.799336639 -705942.72981891;-0.00063 -7.74488310626879e-09 207310.682493421 -705166.202670926;-0.00062 -7.74546140210319e-09 209967.619306521 -704379.653550312;-0.00061 -7.74592961778644e-09 212621.572014987 -703583.093635674;-0.0006 -7.74628774666416e-09 215272.502900276 -702776.53424789;-0.00059 -7.74653578364655e-09 217920.374286791 -701959.986849956;-0.00058 -7.74667372520846e-09 220565.14854242 -701133.463046815;-0.00057 -7.74670156938944e-09 223206.788079066 -700296.974585203;-0.00056 -7.74661931579374e-09 225845.255353184 -699450.53335347;-0.00055 -7.74642696559039e-09 228480.512866314 -698594.151381421;-0.00054 -7.7461245215131e-09 231112.523165613 -697727.840840139;-0.00053 -7.74571198786027e-09 233741.248844389 -696851.614041814;-0.00052 -7.74518937049492e-09 236366.652542632 -695965.483439569;-0.00051 -7.74455667684459e-09 238988.696947543 -695069.461627282;-0.0005 -7.74381391590128e-09 241607.344794067 -694163.561339404;-0.00049 -7.74296109822124e-09 244222.558865423 -693247.795450785;-0.00048 -7.74199823592491e-09 246834.30199363 -692322.176976485;-0.00047 -7.74092534269669e-09 249442.537060036 -691386.719071592;-0.00046 -7.73974243378478e-09 252047.226995849 -690441.435031032;-0.00045 -7.73844952600092e-09 254648.334782658 -689486.338289385;-0.00044 -7.7370466377202e-09 257245.823452964 -688521.442420689;-0.00043 -7.73553378888076e-09 259839.656090704 -687546.76113825;-0.00042 -7.73391100098354e-09 262429.795831774 -686562.308294447;-0.00041 -7.73217829709194e-09 265016.205864556 -685568.097880534;-0.0004 -7.73033570183152e-09 267598.849430438 -684564.144026442;-0.00039 -7.72838324138964e-09 270177.689824338 -683550.461000577;-0.00038 -7.72632094351508e-09 272752.690395225 -682527.063209618;-0.00037 -7.72414883751767e-09 275323.814546643 -681493.965198314;-0.00036 -7.72186695426783e-09 277891.025737225 -680451.181649273;-0.00035 -7.71947532619617e-09 280454.287481219 -679398.72738276;-0.00034 -7.71697398729303e-09 283013.563349 -678336.617356477;-0.00033 -7.71436297310796e-09 285568.816967594 -677264.86666536;-0.00032 -7.71164232074927e-09 288120.012021191 -676183.490541359;-0.00031 -7.70881206888344e-09 290667.112251661 -675092.504353221;-0.0003 -7.70587225773461e-09 293210.081459074 -673991.923606275;-0.00029 -7.70282292908401e-09 295748.883502207 -672881.763942211;-0.00028 -7.69966412626935e-09 298283.482299063 -671762.041138853;-0.00027 -7.69639589418421e-09 300813.841827384 -670632.771109942;-0.00026 -7.69301827927739e-09 ...(+1653 chars)]  x3=[-0.00102 2.59646262568767e-11 0 0;-0.00101 2.63570440024805e-11 0 0;-0.001 2.67490871561476e-11 0 0;-0.00099 2.71407501460769e-11 0 0;-0.00098 2.75320274058705e-11 0 0;-0.00097 2.79229133746124e-11 0 0;-0.00096 2.83134024969476e-11 0 0;-0.00095 2.87034892231616e-11 0 0;-0.00094 2.90931680092583e-11 0 0;-0.00093 2.94824333170398e-11 0 0;-0.00092 2.98712796141843e-11 0 0;-0.00091 3.02597013743252e-11 0 0;-0.0009 3.06476930771296e-11 0 0;-0.00089 3.10352492083766e-11 0 0;-0.00088 3.14223642600356e-11 0 0;-0.00087 3.18090327303449e-11 0 0;-0.00086 3.21952491238896e-11 0 0;-0.00085 3.25810079516799e-11 0 0;-0.00084 3.29663037312291e-11 0 0;-0.00083 3.3351130986631e-11 0 0;-0.00082 3.37354842486388e-11 0 0;-0.00081 3.41193580547418e-11 0 0;-0.0008 3.45027469492434e-11 0 0;-0.00079 3.48856454833388e-11 0 0;-0.00078 3.52680482151924e-11 0 0;-0.00077 3.56499497100148e-11 0 0;-0.00076 3.60313445401404e-11 0 0;-0.00075 3.64122272851046e-11 0 0;-0.00074 3.67925925317204e-11 0 0;-0.00073 3.71724348741558e-11 0 0;-0.00072 3.75517489140102e-11 0 0;-0.00071 3.79305292603915e-11 0 0;-0.0007 3.83087705299926e-11 0 0;-0.00069 3.86864673471678e-11 51.1574027920057 -870.186483604275;-0.00068 3.90636143440093e-11 54.4375245182599 -869.987501939416;-0.00067 3.94402061604235e-11 57.7168725667932 -869.776155826432;-0.00066 3.9816237444207e-11 60.9954003308105 -869.55244826902;-0.00065 4.0191702851123e-11 64.2730612151756 -869.316382446559;-0.00064 4.05665970449769e-11 67.5498086370719 -869.067961714067;-0.00063 4.09409146976925e-11 70.8255960266658 -868.807189602153;-0.00062 4.13146504893872e-11 74.1003768277671 -868.534069816965;-0.00061 4.16877991084483e-11 77.3741044984923 -868.24860624014;-0.0006 4.20603552516079e-11 80.6467325119246 -867.950802928748;-0.00059 4.24323136240186e-11 83.9182143567758 -867.640664115232;-0.00058 4.28036689393285e-11 87.1885035380477 -867.318194207352;-0.00057 4.31744159197567e-11 90.457553577692 -866.983397788119;-0.00056 4.35445492961678e-11 93.7253180152718 -866.636279615731;-0.00055 4.39140638081473e-11 96.991750408621 -866.276844623505;-0.00054 4.42829542040761e-11 100.256804334505 -865.90509791981;-0.00053 4.46512152412051e-11 103.520433389281 -865.521044787987;-0.00052 4.50188416857299e-11 106.782591189555 -865.124690686282;-0.00051 4.53858283128648e-11 110.043231372845 -864.716041247765;-0.0005 4.57521699069177e-11 113.302307598235 -864.295102280248;-0.00049 4.61178612613635e-11 116.559773547039 -863.861879766206;-0.00048 4.64828971789186e-11 119.815582923456 -863.41637986269;-0.00047 4.68472724716147e-11 123.069689455226 -862.958608901238;-0.00046 4.72109819608723e-11 126.322046894294 -862.488573387792;-0.00045 4.75740204775744e-11 129.572609017462 -862.006280002594;-0.00044 4.79363828621403e-11 132.821329627045 -861.511735600102;-0.00043 4.82980639645982e-11 136.068162551534 -861.004947208886;-0.00042 4.86590586446591e-11 139.313061646245 -860.485922031531;-0.00041 4.90193617717897e-11 142.55598079398 -859.954667444534;-0.0004 4.93789682252848e-11 145.79687390568 -859.411190998199;-0.00039 4.97378728943409e-11 149.035694921079 -858.855500416528;-0.00038 5.00960706781281e-11 152.272397809362 -858.287603597116;-0.00037 5.0453556485863e-11 155.506936569816 -857.707508611032;-0.00036 5.08103252368811e-11 158.739265232487 -857.11522370271;-0.00035 5.11663718607086e-11 161.969337858828 -856.510757289831;-0.00034 5.15216912971349e-11 165.197108542358 -855.894117963199;-0.00033 5.18762784962844e-11 168.422531409311 -855.265314486625;-0.00032 5.2230128418688e-11 171.645560619289 -854.624355796798;-0.00031 5.25832360353551e-11 174.866150365912 -853.971251003159;-0.0003 5.29355963278449e-11 178.084254877471 -853.306009387774;-0.00029 5.32872042883377e-11 181.299828417578 -852.628640405198;-0.00028 5.3638054919706e-11 184.512825285815 -851.939153682344;-0.00027 5.39881432355858e-11 187.723199818384 -851.237559018344;-0.00026 5.43374642604471e-11 190.930906388758 -850.523866384412;-0.00025 5.46860130296651e-11 ...(+1567 chars)]  x4=[-0.00102 -9.43211804996896e-11 0 0;-0.00101 -9.46933249069332e-11 0 0;-0.001 -9.50641235124257e-11 0 0;-0.00099 -9.54335710462981e-11 0 0;-0.00098 -9.58016622578832e-11 0 0;-0.00097 -9.61683919157902e-11 0 0;-0.00096 -9.65337548079788e-11 0 0;-0.00095 -9.68977457418335e-11 0 0;-0.00094 -9.72603595442377e-11 0 0;-0.00093 -9.76215910616464e-11 0 0;-0.00092 -9.79814351601602e-11 0 0;-0.00091 -9.83398867255979e-11 0 0;-0.0009 -9.86969406635694e-11 0 0;-0.00089 -9.90525918995479e-11 0 0;-0.00088 -9.9406835378942e-11 0 0;-0.00087 -9.97596660671679e-11 0 0;-0.00086 -1.0011107894972e-10 0 0;-0.00085 -1.00461069032245e-10 0 0;-0.00084 -1.00809631340607e-10 0 0;-0.00083 -1.01156760920965e-10 0 0;-0.00082 -1.01502452839839e-10 0 0;-0.00081 -1.01846702184183e-10 0 0;-0.0008 -1.0218950406145e-10 0 0;-0.00079 -1.02530853599667e-10 0 0;-0.00078 -1.02870745947503e-10 0 0;-0.00077 -1.03209176274333e-10 0 0;-0.00076 -1.03546139770314e-10 0 0;-0.00075 -1.0388163164645e-10 0 0;-0.00074 -1.04215647134657e-10 0 0;-0.00073 -1.04548181487836e-10 0 0;-0.00072 -1.04879229979939e-10 0 0;-0.00071 -1.05208787906032e-10 0 0;-0.0007 -1.0553685058237e-10 0 0;-0.00069 -1.05863413346454e-10 1229.92660311783 -4729.26144347503;-0.00068 -1.06188471557106e-10 1247.74678272859 -4724.59110540767;-0.00067 -1.06512020594527e-10 1265.54922909567 -4719.8536204428;-0.00066 -1.06834055860372e-10 1283.3336892069 -4715.04905591056;-0.00065 -1.07154572777804e-10 1301.09991030575 -4710.17748009445;-0.00064 -1.07473566791571e-10 1318.84763989488 -4705.23896223034;-0.00063 -1.0779103336806e-10 1336.57662573977 -4700.23357250551;-0.00062 -1.08106967995369e-10 1354.28661587229 -4695.16138205763;-0.00061 -1.08421366183367e-10 1371.97735859428 -4690.02246297374;-0.0006 -1.0873422346376e-10 1389.64860248112 -4684.81688828926;-0.00059 -1.09045535390155e-10 1407.30009638533 -4679.54473198693;-0.00058 -1.09355297538118e-10 1424.9315894401 -4674.20606899576;-0.00057 -1.09663505505245e-10 1442.54283106289 -4668.80097518998;-0.00056 -1.09970154911218e-10 1460.13357095898 -4663.32952738792;-0.00055 -1.1027524139787e-10 1477.70355912501 -4657.79180335097;-0.00054 -1.10578760629247e-10 1495.25254585256 -4652.18788178245;-0.00053 -1.10880708291669e-10 1512.78028173168 -4646.51784232649;-0.00052 -1.11181080093791e-10 1530.28651765445 -4640.78176556689;-0.00051 -1.11479871766665e-10 1547.77100481851 -4634.97973302601;-0.0005 -1.117770790638e-10 1565.23349473059 -4629.11182716358;-0.00049 -1.12072697761222e-10 1582.67373921006 -4623.17813137551;-0.00048 -1.12366723657536e-10 1600.09149039244 -4617.17872999277;-0.00047 -1.12659152573982e-10 1617.48650073293 -4611.11370828013;-0.00046 -1.12949980354498e-10 1634.85852300993 -4604.98315243496;-0.00045 -1.13239202865778e-10 1652.20731032855 -4598.78714958605;-0.00044 -1.1352681599733e-10 1669.53261612412 -4592.5257877923;-0.00043 -1.13812815661534e-10 1686.83419416569 -4586.19915604153;-0.00042 -1.14097197793703e-10 1704.11179855955 -4579.80734424917;-0.00041 -1.14379958352136e-10 1721.36518375269 -4573.35044325703;-0.0004 -1.1466109331818e-10 1738.59410453632 -4566.82854483195;-0.00039 -1.14940598696285e-10 1755.79831604934 -4560.24174166455;-0.00038 -1.15218470514061e-10 1772.97757378181 -4553.59012736788;-0.00037 -1.15494704822335e-10 1790.13163357847 -4546.8737964761;-0.00036 -1.15769297695205e-10 1807.26025164215 -4540.09284444315;-0.00035 -1.16042245230098e-10 1824.36318453727 -4533.24736764136;-0.00034 -1.16313543547827e-10 1841.44018919331 -4526.33746336011;-0.00033 -1.16583188792641e-10 1858.49102290822 -4519.36322980443;-0.00032 -1.16851177132285e-10 1875.51544335191 -4512.32476609362;-0.00031 -1.17117504758052e-10 1892.51320856969 -4505.22217225983;-0.0003 -1.17382167884835e-10 1909.48407698568 -4498.05554924664;-0.00029 -1.17645162751187e-10 1926.42780740629 -4490.82499890762;-0.00028 -1.17906485619368e-10 1943.3441590236 -4483.53062400491;-0.00027 -1.18166132775401e-10 1960.23289141881 -4476.17252820771;-0.00026 -1.18424100529127e-10 ...(+1657 chars)]  x5=0.00101545182061977  V1=ones(3,3)  V2=ones(3,3)  I1=ones(3,3)  I2=ones(3,3)  nHarmo=1  Measurements=None  Decoupling=off  VsMag0=0  VrMag0=0  VsAngle0=0  VrAngle0=0  IsMag0=0  IrMag0=0  IsAngle0=0  IrAngle0=0
      settings: AttributesFormatString=\n
  200 MW : spsThreePhaseSeriesRLCLoadLib/Three-Phase Series RLC Load  LConnTagsString=A|B|C  Configuration=Y (grounded)  NominalVoltage=13.8e3  Vabc=[1e3 1e3 1e3]  Vabcp=[1e3 1e3 1e3]  NominalFrequency=60  UnbalancedPower=off  ActivePower=2e+008  InductivePower=0  CapacitivePower=0  Pabc=[10e3 9e3 11e3]  QLabc=[100 90 110]  QCabc=[100 90 110]  Pabcp=[10e3 9e3 11e3]  QLabcp=[100 90 110]  QCabcp=[100 90 110]  Measurements=None  LoadType=constant Z
  200 Mvar with L neutral : Subsystem
  "200 Mvar with L neutral " : Subsystem
  200 Mvar1 : spsThreePhaseSeriesRLCLoadLib/Three-Phase Series RLC Load  LConnTagsString=A|B|C  Configuration=Y (grounded)  NominalVoltage=735e3  Vabc=[1e3 1e3 1e3]  Vabcp=[1e3 1e3 1e3]  NominalFrequency=60  UnbalancedPower=off  ActivePower=800000  InductivePower=200e6  CapacitivePower=0  Pabc=[10e3 9e3 11e3]  QLabc=[100 90 110]  QCabc=[100 90 110]  Pabcp=[10e3 9e3 11e3]  QLabcp=[100 90 110]  QCabcp=[100 90 110]  Measurements=None  LoadType=constant Z
  200 Mvar2 : spsThreePhaseSeriesRLCLoadLib/Three-Phase Series RLC Load  LConnTagsString=A|B|C  Configuration=Y (grounded)  NominalVoltage=735e3  Vabc=[1e3 1e3 1e3]  Vabcp=[1e3 1e3 1e3]  NominalFrequency=60  UnbalancedPower=off  ActivePower=800000  InductivePower=200e6  CapacitivePower=0  Pabc=[10e3 9e3 11e3]  QLabc=[100 90 110]  QCabc=[100 90 110]  Pabcp=[10e3 9e3 11e3]  QLabcp=[100 90 110]  QCabcp=[100 90 110]  Measurements=None  LoadType=constant Z
  Arc  Model : Subsystem  mask(Arc model){Rarc_var=off, Rarc_fixed=0, Rparam=[56.54 0.006375], I0=200, Ts=1e-5}
      mask prompts: Rarc_var "Variable arc resistance :"; Rarc_fixed "Arc resistance for fixed arc resistance :"; Rparam "Arc parameters for variable arc resistance [Ro k] : :"; I0 "Current threshold for arc extinction Io (A rms) :"; Ts "Sample time (s) :"
      mask help:
      | This block implements a variable or fixed arc resistance model.
      |
      | Input 1, output 1:  Connection terminals of the arc resistance.
      | Input 2 :    Control signal for the fault initiation
      | Use a short pulse of 1 cycle. Once fault current starts flowing, it is sustained by the arc ionized path.
      | Output 2:  Arc resitance
      |
      | If you check the 'Variable arc resistance' box, the mean arc resistance will be a function of the arc current, according to equation below. Otherwise, the resistance will be kept constant.
      |
      |        Rarc= Ro*exp(-k*i)
      |
      | where:   i = rms value of the arc current (A)
      |              Ro, k = arc parameters
      |
      | The arc extinguishes at the next zero current crossing after its  rms value has fallen  below  the specified threshold current Io.
      mask init:
      | if strcmp(Rarc_var,'on'), rvar=1; else, rvar=0; end
      | R0=Rparam(1);
      | k=Rparam(2);
  Cast To Boolean : DataTypeConversion  OutDataTypeStr=boolean  SaturateOnIntegerOverflow=off  RndMeth=Floor
  Demux : Demux  Outputs=3
  Demux1 : Demux  Outputs=3
  Display1 : Display
  Display8 : Display
  Fault initiation : spsStairGeneratorLib/Stair Generator  t=[0.2 0.75]  e=[1 0]  Ts=1e-5
  Filter : Subsystem
  Filter1 : Subsystem
  Ground : spsGroundLib/Ground  LConnTagsString=a
  Lamp : LampBlock  LabelPosition=Hide
  Load Flow Bus : spsLoadFlowBusLib/Load Flow Bus  LConnTagsString=a  Phases=single  Connectors=on one side  ID=B1  Vbase=735e3  Vref=1  Vangle=0  VLF=0.9936  VLFb=1  VLFc=1  angleLF=10.42  angleLFb=0  angleLFc=0
      settings: AttributesFormatString=%<ID>\n%<Vbase>V\n%<VLF>pu\n%<angleLF>deg.
  Load Flow Bus1 : spsLoadFlowBusLib/Load Flow Bus  LConnTagsString=a  Phases=single  Connectors=on one side  ID=B2  Vbase=735e3  Vref=1  Vangle=0  VLF=1  VLFb=1  VLFc=1  angleLF=0  angleLFb=0  angleLFc=0
      settings: AttributesFormatString=%<ID>\n%<Vbase>V\n%<VLF>pu\n%<angleLF>deg.
  Load Flow Bus2 : spsLoadFlowBusLib/Load Flow Bus  LConnTagsString=a  Phases=single  Connectors=on one side  ID=GEN  Vbase=13.8e3  Vref=1  Vangle=0  VLF=1  VLFb=1  VLFc=1  angleLF=-12.96  angleLFb=0  angleLFc=0
      settings: AttributesFormatString=%<ID>\n%<Vbase>V\n%<VLF>pu\n%<angleLF>deg.
  Load Flow Bus3 : spsLoadFlowBusLib/Load Flow Bus  LConnTagsString=a  Phases=single  Connectors=on one side  ID=B3  Vbase=735e3  Vref=1  Vangle=0  VLF=1.001  VLFb=1  VLFc=1  angleLF=5.175  angleLFb=0  angleLFc=0
      settings: AttributesFormatString=%<ID>\n%<Vbase>V\n%<VLF>pu\n%<angleLF>deg.
  More Info : Subsystem
      settings: OpenFcn="showExample(\"simscapeelectricalsps/SinglePoleLineReclosingExample\")"
      mask Display: disp('?')
  N1 : spsThreePhaseVIMeasurementLib/Three-Phase V-I Measurement  VoltageMeasurement=phase-to-ground  SetLabelV=on  LabelV=VN1  Vpu=on  VpuLL=off  CurrentMeasurement=yes  SetLabelI=on  LabelI=IN1  Ipu=on  Pbase=100e6  Vbase=735e3  OutputType=Magnitude  PhasorSimulation=off  PSBequivalent=0
  N2 : spsThreePhaseVIMeasurementLib/Three-Phase V-I Measurement  VoltageMeasurement=phase-to-ground  SetLabelV=on  LabelV=VN2  Vpu=on  VpuLL=off  CurrentMeasurement=yes  SetLabelI=on  LabelI=IN2  Ipu=on  Pbase=100e6  Vbase=735e3  OutputType=Magnitude  PhasorSimulation=off  PSBequivalent=0
  N2B : spsThreePhaseBreakerLib/Three-Phase Breaker  InitialState=closed  SwitchA=off  SwitchB=off  SwitchC=off  SwitchTimes="[4/60  34/60]"  External=off  BreakerResistance=0.001  SnubberResistance=1e5  SnubberCapacitance=inf  Measurements=None
      settings: AttributesFormatString=\n
  N3 : spsThreePhaseVIMeasurementLib/Three-Phase V-I Measurement  VoltageMeasurement=phase-to-ground  SetLabelV=on  LabelV=VN3  Vpu=on  VpuLL=off  CurrentMeasurement=yes  SetLabelI=on  LabelI=IN3  Ipu=on  Pbase=100e6  Vbase=735e3  OutputType=Magnitude  PhasorSimulation=off  PSBequivalent=0
  N4 : spsThreePhaseVIMeasurementLib/Three-Phase V-I Measurement  VoltageMeasurement=phase-to-ground  SetLabelV=on  LabelV=VN4  Vpu=on  VpuLL=off  CurrentMeasurement=yes  SetLabelI=on  LabelI=IN4  Ipu=on  Pbase=100e6  Vbase=735e3  OutputType=Magnitude  PhasorSimulation=off  PSBequivalent=0
  "Overcurrent Relay End 1 " : Subsystem
  Overcurrent Relay End 2 : Subsystem
  Pmec (pu) : Constant  Value=0.775349
  Pulse Generator : DiscretePulseGenerator  PulseType=Time based  Period=[0.4]
  Scope : Scope  NumInputPorts=4
  Scope{1..4} (4 alike) : Scope
  Terminator : Terminator
  To Workspace : ToWorkspace  VariableName=VN3  SaveFormat=Timeseries  SampleTime=-1
  To Workspace1 : ToWorkspace  VariableName=IN3  SaveFormat=Timeseries  SampleTime=-1
  To Workspace2 : ToWorkspace  VariableName=VN4  SaveFormat=Timeseries  SampleTime=-1
  To Workspace3 : ToWorkspace  VariableName=IN4  SaveFormat=Timeseries  SampleTime=-1
  To Workspace4 : ToWorkspace  VariableName=VN1  SaveFormat=Timeseries  SampleTime=-1
  To Workspace5 : ToWorkspace  VariableName=IN1  SaveFormat=Timeseries  SampleTime=-1
  To Workspace6 : ToWorkspace  VariableName=VN2  SaveFormat=Timeseries  SampleTime=-1
  To Workspace7 : ToWorkspace  VariableName=IN2  SaveFormat=Timeseries  SampleTime=-1
  Vfield (pu) : Constant  Value=1.0391
  W1 : spsThreePhaseBreakerLib/Three-Phase Breaker  InitialState=closed  SwitchA=off  SwitchB=off  SwitchC=off  SwitchTimes="[4/60  34/60]"  External=off  BreakerResistance=0.001  SnubberResistance=1e5  SnubberCapacitance=inf  Measurements=Breaker voltages and currents
      settings: AttributesFormatString=\n
  powergui : spspowerguiLib/powergui  Priority=2  SimulationMode=Discrete  SampleTime=1e-5  frequency=60  Iterations=50  frequencyindice=0  Pbase=100e6  ErrMax=0.0001  UnitsV=kV  UnitsW=MW  buscounter=0  FunctionMessages=off  echomessages=off  EnableUseOfTLC=off  CurrentSourceSwitches=off  DisableSnubberDevices=off  DisableRonSwitches=off  DisableVfSwitches=off  DisplayEquations=off  AutomaticDiscreteSolvers=off  SolverType=Tustin/Backward Euler (TBE)  Interpol=off  ExternalGateDelay=off  methode=off  Ts=0  x0status=blocks  SPID=off  SwTol=0  HookPort=off  NonlinearTolerance=1e-4  nMaxIteration=100  ContinueOnMaxIteration=off  RestoreLinks=warning  ResistiveCurrentMeasurement=off  Frange=logspace(0,3,50)  Ylog=off  Xlog=off  ShowGrid=off  save=off  variable=ZData  structure=0  ZoomFFT=on  StartTime=0.0  cycles=1  DisplayStyle=off  fundamental=60  FreqAxis=off  MaxFrequency=1000  frequencyindicesteady=1  RmsSteady=1  display=off
  wires:
  Fault initiation/1 -> Scope2/1, Arc  Model/1(fault_init)
  Arc  Model/1(R_arc) -> Scope/1  "R_arc (ohms)"
  Vfield (pu)/1 -> 12*350 MVA Generators/2
  Pmec (pu)/1 -> 12*350 MVA Generators/1
  12*350 MVA Generators/1 -> Terminator/1
  Arc  Model/2(i_arc) -> Scope/2  "i arc (A)"
  [VN3] -> Scope/3
  [IN3] -> Scope/4
  Demux/2 -> Filter/2(In4)
  Demux/1 -> Filter/1(In2)
  Demux/3 -> Filter/3(In6)
  [IN3] -> Demux/1
  Filter/1(I1) -> "Overcurrent Relay End 1 "/2(I1)
  Filter/2(I2) -> "Overcurrent Relay End 1 "/3(I2)
  Filter/3(I3) -> "Overcurrent Relay End 1 "/4(I3)
  [VN3] -> To Workspace/1
  [IN3] -> To Workspace1/1
  [VN4] -> To Workspace2/1
  [IN4] -> To Workspace3/1
  [IN2] -> To Workspace7/1
  [VN1] -> To Workspace4/1
  [VN2] -> To Workspace6/1
  [IN1] -> To Workspace5/1
  [IN4] -> Demux1/1
  Filter1/3(I3) -> Overcurrent Relay End 2/3(I3)
  Demux1/2 -> Filter1/2(In4)
  Demux1/1 -> Filter1/1(In2)
  Filter1/2(I2) -> Overcurrent Relay End 2/2(I2)
  Demux1/3 -> Filter1/3(In6)
  Filter1/1(I1) -> Overcurrent Relay End 2/1(I1)
  [D_50_E2] -> "  N4B"/1
  [D_50_E1] -> "  N3B"/1
  Overcurrent Relay End 2/1(Tripping Signal) -> [D_50_E2], Display1/1, Scope1/1
  "Overcurrent Relay End 1 "/1(Tripping Signal) -> [D_50_E1], Display8/1, Scope3/1
  Cast To Boolean/1 -> "Overcurrent Relay End 1 "/1(R), Overcurrent Relay End 2/4(R)
  Pulse Generator/1 -> Cast To Boolean/1
  connections:
  "100  km "/LConn3 -- "  N3B"/RConn3 -- "200 Mvar with L neutral "/LConn3
  "100  km  "/RConn1 -- "  N4B"/LConn1 -- 200 Mvar with L neutral/LConn1
  "100  km  "/RConn2 -- "  N4B"/LConn2 -- 200 Mvar with L neutral/LConn2
  "100  km  "/RConn3 -- "  N4B"/LConn3 -- 200 Mvar with L neutral/LConn3
  20,000 MVA 735 kV equivalent/RConn1 -- N2B/RConn1 -- N4/RConn1
  20,000 MVA 735 kV equivalent/RConn2 -- N4/RConn2 -- N2B/RConn2
  N2B/RConn3 -- Load Flow Bus1/LConn1 -- N4/RConn3 -- 20,000 MVA 735 kV equivalent/RConn3
  "100  km "/LConn1 -- "  N3B"/RConn1 -- "200 Mvar with L neutral "/LConn1
  "100  km "/LConn2 -- "  N3B"/RConn2 -- "200 Mvar with L neutral "/LConn2
  12*350 MVA Generators/RConn2 -- 200 MW/LConn2 -- W1/LConn2
  12*350 MVA Generators/RConn1 -- Load Flow Bus2/LConn1 -- W1/LConn1 -- 200 MW/LConn1
  12*350 MVA Generators/RConn3 -- 200 MW/LConn3 -- W1/LConn3
  N1/RConn1 -- 200 Mvar1/LConn1 -- 200  km/LConn1
  " W2"/RConn2 -- N3/LConn2 -- " N1B"/LConn2
  " W2"/RConn3 -- N3/LConn3 -- Load Flow Bus/LConn1 -- " N1B"/LConn3
  " W2"/RConn1 -- N3/LConn1 -- " N1B"/LConn1
  N1/RConn2 -- 200 Mvar1/LConn2 -- 200  km/LConn2
  200  km/LConn3 -- 200 Mvar1/LConn3 -- N1/RConn3
  200 Mvar2/LConn1 -- N2/LConn1 -- 200  km/RConn1
  200 Mvar2/LConn2 -- N2/LConn2 -- 200  km/RConn2
  200 Mvar2/LConn3 -- N2/LConn3 -- 200  km/RConn3
  " N1B"/RConn1 -- N1/LConn1
  " N1B"/RConn2 -- N1/LConn2
  " N1B"/RConn3 -- N1/LConn3
  N2/RConn1 -- N2B/LConn1
  N2/RConn2 -- N2B/LConn2
  N2/RConn3 -- N2B/LConn3
  12*350 MVA 13.8/735 kV/RConn1 -- " W2"/LConn1
  12*350 MVA 13.8/735 kV/RConn2 -- " W2"/LConn2
  12*350 MVA 13.8/735 kV/RConn3 -- " W2"/LConn3
  12*350 MVA 13.8/735 kV/LConn1 -- W1/RConn1
  W1/RConn2 -- 12*350 MVA 13.8/735 kV/LConn2
  W1/RConn3 -- 12*350 MVA 13.8/735 kV/LConn3
  "100  km "/RConn1 -- Arc  Model/LConn1 -- "100  km  "/LConn1
  "100  km  "/LConn3 -- "100  km "/RConn3 -- Load Flow Bus3/LConn1
  Ground/LConn1 -- Arc  Model/RConn1
  "100  km "/RConn2 -- "100  km  "/LConn2
  "  N3B"/LConn2 -- N3/RConn2
  "  N3B"/LConn3 -- N3/RConn3
  N4/LConn1 -- "  N4B"/RConn1
  N4/LConn2 -- "  N4B"/RConn2
  N4/LConn3 -- "  N4B"/RConn3
  N3/RConn1 -- "  N3B"/LConn1
